simulink model "ACC_System_Closed_Loop"  (R2024b)
settings: Solver=ode3  StartTime=0.0  StopTime=10.0  FixedStep=0.01  RelTol=1e-3
InitFcn:
  | init_params; import_fusion_data;
undefined symbols (not defined in the file or in its folder): A_front, Cd, d_safe_min, default_time_gap, eff_drive, f_roll, g, ig, Jm, Jw, m, max_brake_torque, rho_air, rw
settings Model: Creator=ezers  LastModifiedBy=ezers

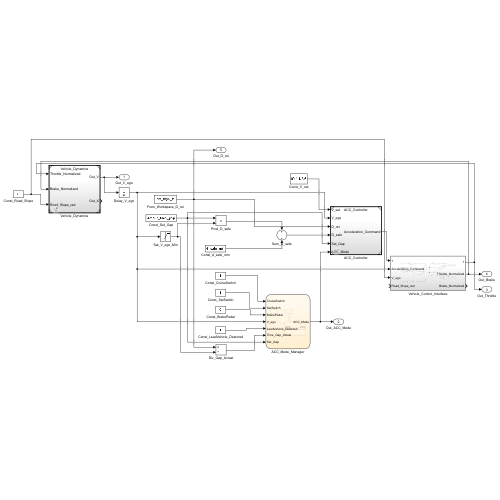
[thumbnail: Simulink's stored preview of the top-level diagram]
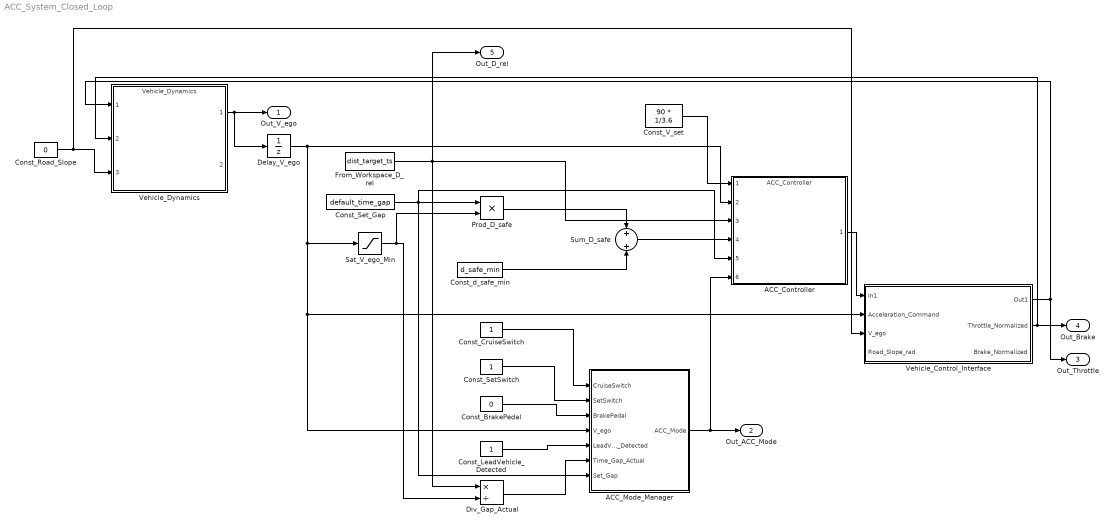
== system ACC_System_Closed_Loop ==
  ACC_Controller : ModelReference  ModelNameDialog=ACC_Controller  SimulationMode=Normal  ModelReferenceVersion=1.14
  ACC_Mode_Manager : Stateflow chart  TreatAsAtomicUnit=on
  Const_BrakePedal : Constant  Value=0  OutDataTypeStr=boolean
  Const_CruiseSwitch : Constant  OutDataTypeStr=boolean
  Const_LeadVehicle_Detected : Constant  OutDataTypeStr=boolean
  Const_Road_Slope : Constant  Value=0
  Const_SetSwitch : Constant  OutDataTypeStr=boolean
  Const_Set_Gap : Constant  Value=default_time_gap
  Const_V_set : Constant  Value=90 * 1/3.6
  Const_d_safe_min : Constant  Value=d_safe_min
  Delay_V_ego : UnitDelay  SampleTime=0.01  HasFrameUpgradeWarning=on
  Div_Gap_Actual : Product  Inputs=*/
  From_Workspace_D_rel : FromWorkspace  VariableName=dist_target_ts
  Prod_D_safe : Product
  Sat_V_ego_Min : Saturate  UpperLimit=100  LowerLimit=0.5
  Sum_D_safe : Sum
  Vehicle_Control_Interface : Subsystem
  Vehicle_Dynamics : ModelReference  ModelNameDialog=Vehicle_Dynamics  SimulationMode=Normal  ModelReferenceVersion=1.5
  Out_V_ego : Outport
  Out_ACC_Mode : Outport  Port=2
  Out_Throttle : Outport  Port=3
  Out_Brake : Outport  Port=4
  Out_D_rel : Outport  Port=5
  wires:
  Const_CruiseSwitch/1 -> ACC_Mode_Manager/1(CruiseSwitch)
  Const_Road_Slope/1 -> Vehicle_Control_Interface/3(V_ego), Vehicle_Dynamics/3
  Const_Set_Gap/1 -> ACC_Mode_Manager/7(Set_Gap), Prod_D_safe/1, ACC_Controller/5
  Const_d_safe_min/1 -> Sum_D_safe/2
  From_Workspace_D_rel/1 -> ACC_Controller/3, Out_D_rel/1, Div_Gap_Actual/1
  Div_Gap_Actual/1 -> ACC_Mode_Manager/6(Time_Gap_Actual)
  Delay_V_ego/1 -> ACC_Mode_Manager/4(V_ego), Vehicle_Control_Interface/2(Acceleration_Command), Sat_V_ego_Min/1, ACC_Controller/2
  Vehicle_Dynamics/1 -> Out_V_ego/1, Delay_V_ego/1
  Prod_D_safe/1 -> Sum_D_safe/1
  Sum_D_safe/1 -> ACC_Controller/4
  Sat_V_ego_Min/1 -> Div_Gap_Actual/2, Prod_D_safe/2
  Const_V_set/1 -> ACC_Controller/1
  Const_LeadVehicle_Detected/1 -> ACC_Mode_Manager/5(LeadVehicle_Detected)
  Const_SetSwitch/1 -> ACC_Mode_Manager/2(SetSwitch)
  Const_BrakePedal/1 -> ACC_Mode_Manager/3(BrakePedal)
  ACC_Mode_Manager/1(ACC_Mode) -> ACC_Controller/6, Out_ACC_Mode/1
  ACC_Controller/1 -> Vehicle_Control_Interface/1(In1)
  Vehicle_Control_Interface/1(Out1) -> Vehicle_Dynamics/1, Out_Throttle/1
  Vehicle_Control_Interface/2(Throttle_Normalized) -> Vehicle_Dynamics/2, Out_Brake/1

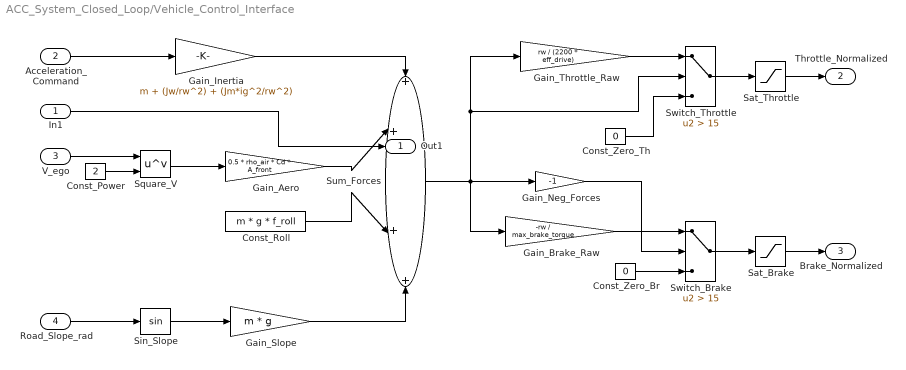
== system ACC_System_Closed_Loop/Vehicle_Control_Interface ==
  In1 : Inport
  Acceleration_Command : Inport  Port=2
  V_ego : Inport  Port=3
  Road_Slope_rad : Inport  Port=4
  Const_Power : Constant  Value=2
  Const_Roll : Constant  Value=m * g * f_roll
  Const_Zero_Br : Constant  Value=0
  Const_Zero_Th : Constant  Value=0
  Gain_Aero : Gain  Gain=0.5 * rho_air * Cd * A_front
  Gain_Brake_Raw : Gain  Gain=-rw / max_brake_torque
  Gain_Inertia : Gain  Gain=m + (Jw/rw^2) + (Jm*ig^2/rw^2)
  Gain_Neg_Forces : Gain  Gain=-1
  Gain_Slope : Gain  Gain=m * g
  Gain_Throttle_Raw : Gain  Gain=rw / (2200 * eff_drive)
  Sat_Brake : Saturate  UpperLimit=1  LowerLimit=0
  Sat_Throttle : Saturate  UpperLimit=1  LowerLimit=0
  Sin_Slope : Trigonometry
  Square_V : Math  Operator=pow
  Sum_Forces : Sum  Inputs=++++
  Switch_Brake : Switch  Criteria=u2 > Threshold  Threshold=15  SaturateOnIntegerOverflow=off  InputSameDT=off
  Switch_Throttle : Switch  Criteria=u2 > Threshold  Threshold=15  SaturateOnIntegerOverflow=off  InputSameDT=off
  Out1 : Outport
  Throttle_Normalized : Outport  Port=2
  Brake_Normalized : Outport  Port=3
  wires:
  In1/1 -> Out1/1
  Acceleration_Command/1 -> Gain_Inertia/1
  V_ego/1 -> Square_V/1
  Const_Power/1 -> Square_V/2
  Square_V/1 -> Gain_Aero/1
  Road_Slope_rad/1 -> Sin_Slope/1
  Sin_Slope/1 -> Gain_Slope/1
  Gain_Inertia/1 -> Sum_Forces/1
  Gain_Aero/1 -> Sum_Forces/2
  Const_Roll/1 -> Sum_Forces/3
  Gain_Slope/1 -> Sum_Forces/4
  Sum_Forces/1 -> Gain_Throttle_Raw/1, Switch_Throttle/2, Gain_Neg_Forces/1, Gain_Brake_Raw/1
  Gain_Throttle_Raw/1 -> Switch_Throttle/1
  Const_Zero_Th/1 -> Switch_Throttle/3
  Gain_Brake_Raw/1 -> Switch_Brake/1
  Gain_Neg_Forces/1 -> Switch_Brake/2
  Const_Zero_Br/1 -> Switch_Brake/3
  Switch_Throttle/1 -> Sat_Throttle/1
  Switch_Brake/1 -> Sat_Brake/1
  Sat_Throttle/1 -> Throttle_Normalized/1
  Sat_Brake/1 -> Brake_Normalized/1

== stateflow chart ACC_System_Closed_Loop/ACC_Mode_Manager ==
  state ACC_STANDBY
    entry: ACC_Mode = 1;
  state ACC_OFF
    entry: ACC_Mode = 0;
  state ACC_ACTIVE
    state Speed_Control
      entry: ACC_Mode = 2;
    state Gap_Control
      entry: ACC_Mode = 3;
    (default) -> Speed_Control
    Gap_Control -> Speed_Control : [LeadVehicle_Detected == true && Time_Gap_Actual < Set_Gap]
    Speed_Control -> Gap_Control : [LeadVehicle_Detected == false || Time_Gap_Actual >= (Set_Gap * 1.2)]
  (default) -> ACC_OFF
  ACC_OFF -> ACC_STANDBY : [CruiseSwitch == true]
  ACC_ACTIVE -> ACC_OFF [order 2] : [CruiseSwitch == false]
  ACC_STANDBY -> ACC_ACTIVE : [SetSwitch == true && BrakePedal == false && V_ego >= 11.11]
  ACC_ACTIVE -> ACC_STANDBY [order 1] : [BrakePedal == true]
  data: CruiseSwitch input boolean; SetSwitch input boolean; BrakePedal input boolean; V_ego input double; LeadVehicle_Detected input boolean; Time_Gap_Actual input double; Set_Gap input double; ACC_Mode output uint8
  data CruiseSwitch settings: description=Bouton Master ON/OFF
  data SetSwitch settings: description=Bouton d'activation de la consigne
  data BrakePedal settings: description=État pédale de frein
  data V_ego settings: description=Vitesse véhicule hôte
  data LeadVehicle_Detected settings: description=Signal de présence (IA Perception)
  data Time_Gap_Actual settings: description=Temps inter-véhiculaire mesuré
  data Set_Gap settings: description=Consigne de sécurité (temps)
